simulink model "surgicalControl_Shared_memory_loop_2015b"  (R2015b)
settings: Solver=FixedStepAuto  SolverMode=SingleTasking  StartTime=0.0  StopTime=inf  FixedStep=1/100  RelTol=1e-3
libraries: dspsigops x9, simulink x3, matlabGenericSHM_Block x1
settings Model: Creator=daniel  LastModifiedBy=migf1
settings DataIOCC: LimitDataPoints=off
settings DebuggingCC: AllowSymbolicDim=on  SFUnexpectedBacktrackingDiag=error  SFNoUnconditionalDefaultTransitionDiag=error
settings ModelReferenceCC: PropagateSignalLabelsOutOfModel=on
settings GRTTargetCC: TargetLangStandard=C99 (ISO)
settings ConfigComp: CovMetricSettings=dwe  CovHtmlReporting=off  CovSaveCumulativeToWorkspaceVar=off  CovSaveSingleToWorkspaceVar=off  CovModelRefEnable=Off  CovExternalEMLEnable=on

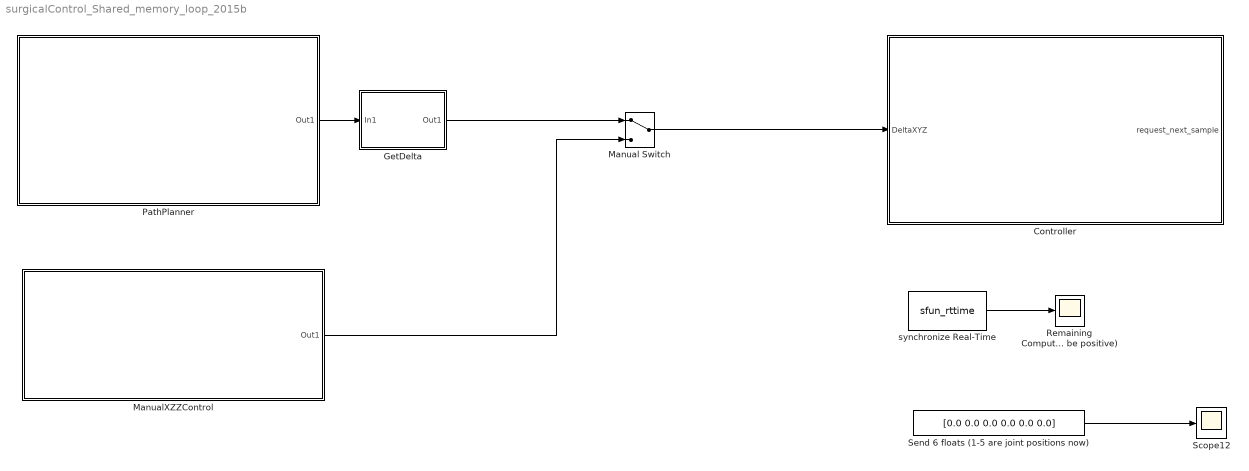
== system surgicalControl_Shared_memory_loop_2015b ==
  " GetDelta " : Subsystem
  Controller : Subsystem
  Manual Switch : ManualSwitch
  "ManualXZZControl " : Subsystem
  PathPlanner : Subsystem
  Remaining Computation Time (must be positive) : Scope
  Scope12 : Scope
  Send 6 floats (1-5 are joint positions now) : Constant  Value=[0.0 0.0 0.0 0.0 0.0 0.0]  OutDataTypeStr=single
  synchronize Real-Time : S-Function  FunctionName=sfun_rttime  Parameters=1  SFunctionDeploymentMode=off  EnableBusSupport=off
  wires:
  synchronize Real-Time/1 -> Remaining Computation Time (must be positive)/1
  Send 6 floats (1-5 are joint positions now)/1 -> Scope12/1
  Manual Switch/1 -> Controller/1(DeltaXYZ)
  PathPlanner/1(Out1) -> " GetDelta "/1(In1)
  "ManualXZZControl "/1(Out1) -> Manual Switch/2
  " GetDelta "/1(Out1) -> Manual Switch/1

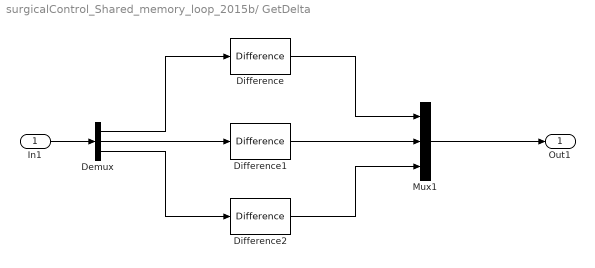
== system surgicalControl_Shared_memory_loop_2015b/ GetDelta  ==
  In1 : Inport
  Demux : Demux  Outputs=3
  Difference : simulink/Discrete/Difference  ICPrevInput=0  OutMin=[]  OutMax=[]  OutDataType=fixdt(1, 16)  OutScaling=2^-10  DoSatur=off
  Difference1 : simulink/Discrete/Difference  ICPrevInput=0  OutMin=[]  OutMax=[]  OutDataType=fixdt(1, 16)  OutScaling=2^-10  DoSatur=off
  Difference2 : simulink/Discrete/Difference  ICPrevInput=0  OutMin=[]  OutMax=[]  OutDataType=fixdt(1, 16)  OutScaling=2^-10  DoSatur=off
  Mux1 : Mux  Inputs=3
  Out1 : Outport
  wires:
  In1/1 -> Demux/1
  Demux/1 -> Difference/1
  Demux/2 -> Difference1/1
  Demux/3 -> Difference2/1
  Difference1/1 -> Mux1/2
  Difference/1 -> Mux1/1
  Difference2/1 -> Mux1/3
  Mux1/1 -> Out1/1

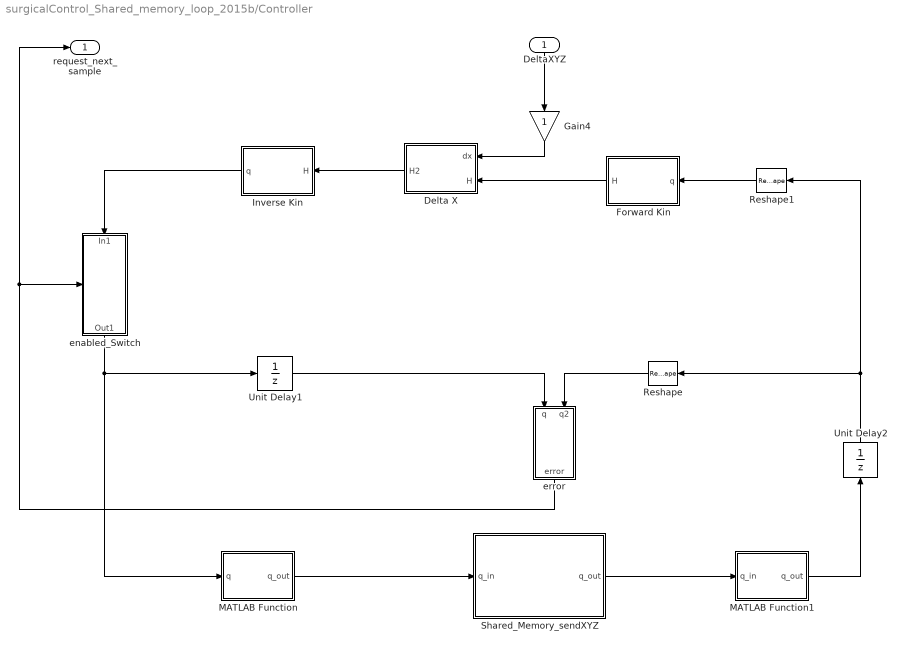
== system surgicalControl_Shared_memory_loop_2015b/Controller ==
  DeltaXYZ : Inport
  Delta X : MATLAB Function  TreatAsAtomicUnit=on
      settings: PermitHierarchicalResolution=ParametersOnly
  Forward Kin : MATLAB Function  TreatAsAtomicUnit=on
      settings: PermitHierarchicalResolution=ParametersOnly
  Gain4 : Gain
  Inverse Kin : MATLAB Function  TreatAsAtomicUnit=on
      settings: PermitHierarchicalResolution=ParametersOnly
  MATLAB Function : MATLAB Function  TreatAsAtomicUnit=on
      settings: PermitHierarchicalResolution=ParametersOnly
  MATLAB Function1 : MATLAB Function  TreatAsAtomicUnit=on
      settings: PermitHierarchicalResolution=ParametersOnly
  Reshape : Reshape
  Reshape1 : Reshape  OutputDimensionality=Customize  OutputDimensions=[1,6]
  Shared_Memory_sendXYZ : Subsystem  mask{ID1=4}
  Unit Delay1 : UnitDelay  InitialCondition=[0.0 0.0 0.0 0.0 0.0 0.0]  SampleTime=-1
  Unit Delay2 : UnitDelay  InitialCondition=[0.0 0.0 0.0 0.0 0.0 0.0]  SampleTime=-1
  "enabled_Switch " : Subsystem  TreatAsAtomicUnit=on
  error : MATLAB Function  TreatAsAtomicUnit=on
      settings: PermitHierarchicalResolution=ParametersOnly
  request_next_sample : Outport
  wires:
  Reshape/1 -> error/2(q2)
  MATLAB Function1/1(q_out) -> Unit Delay2/1
  Shared_Memory_sendXYZ/1(q_out) -> MATLAB Function1/1(q_in)
  Gain4/1 -> Delta X/1(dx)
  Forward Kin/1(H) -> Delta X/2(H)
  DeltaXYZ/1 -> Gain4/1
  Reshape1/1 -> Forward Kin/1(q)
  Unit Delay2/1 -> Reshape/1, Reshape1/1
  "enabled_Switch "/1(Out1) -> Unit Delay1/1, MATLAB Function/1(q)
  MATLAB Function/1(q_out) -> Shared_Memory_sendXYZ/1(q_in)
  error/1(error) -> request_next_sample/1, "enabled_Switch "/Enable
  Unit Delay1/1 -> error/1(q)
  Delta X/1(H2) -> Inverse Kin/1(H)
  Inverse Kin/1(q) -> "enabled_Switch "/1(In1)

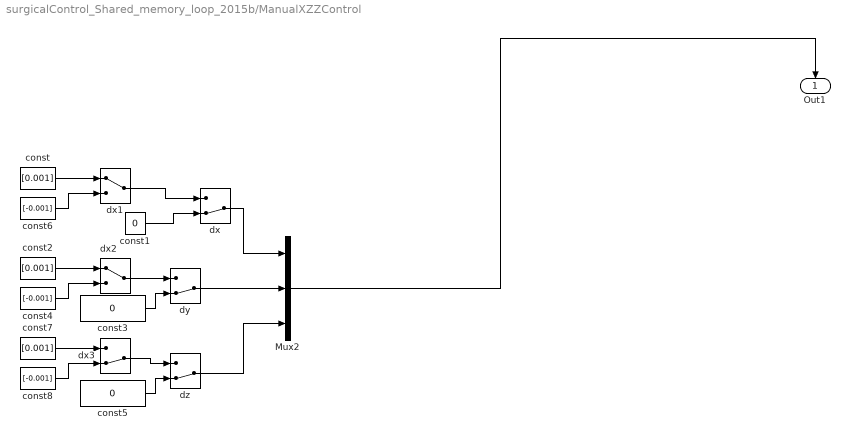
== system surgicalControl_Shared_memory_loop_2015b/ManualXZZControl  ==
  Mux2 : Mux  Inputs=3
  const : Constant  Value=[0.001]  OutDataTypeStr=single
  const1 : Constant  Value=0  OutDataTypeStr=single
  const2 : Constant  Value=[0.001]  OutDataTypeStr=single
  const3 : Constant  Value=0  OutDataTypeStr=single
  const4 : Constant  Value=[-0.001]  OutDataTypeStr=single
  const5 : Constant  Value=0  OutDataTypeStr=single
  const6 : Constant  Value=[-0.001]  OutDataTypeStr=single
  const7 : Constant  Value=[0.001]  OutDataTypeStr=single
  const8 : Constant  Value=[-0.001]  OutDataTypeStr=single
  dx : ManualSwitch  CurrentSetting=0
  dx1 : ManualSwitch
  dx2 : ManualSwitch
  dx3 : ManualSwitch  CurrentSetting=0
  dy : ManualSwitch  CurrentSetting=0
  dz : ManualSwitch  CurrentSetting=0
  Out1 : Outport
  wires:
  const/1 -> dx1/1
  const6/1 -> dx1/2
  const2/1 -> dx2/1
  dz/1 -> Mux2/3
  dx/1 -> Mux2/1
  dx2/1 -> dy/1
  dy/1 -> Mux2/2
  dx3/1 -> dz/1
  const5/1 -> dz/2
  Mux2/1 -> Out1/1
  const8/1 -> dx3/2
  const7/1 -> dx3/1
  const3/1 -> dy/2
  const1/1 -> dx/2
  dx1/1 -> dx/1
  const4/1 -> dx2/2

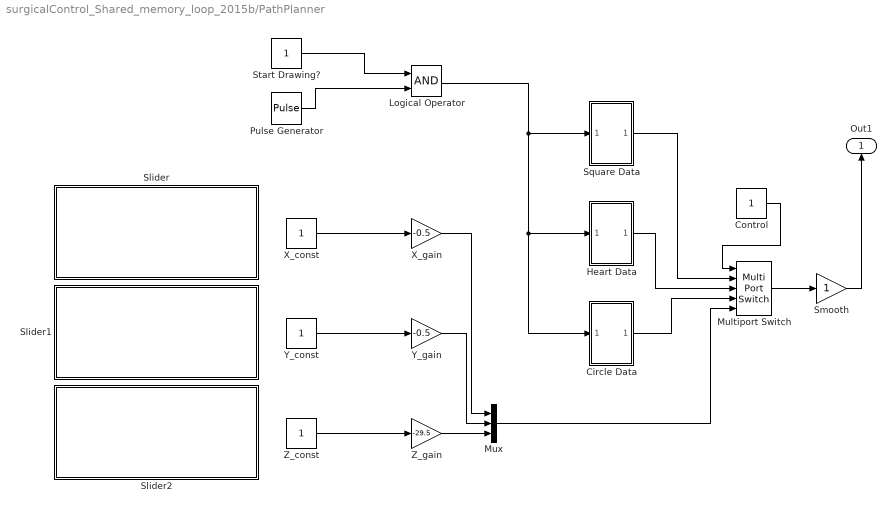
== system surgicalControl_Shared_memory_loop_2015b/PathPlanner ==
  " X_const " : Constant
  " Y_const" : Constant
  " Z_const" : Constant
  Circle Data : Subsystem
  "Control " : Constant
  Heart Data : Subsystem
  Logical Operator : Logic  AllPortsSameDT=off  OutDataTypeStr=boolean
  Multiport Switch : MultiPortSwitch  Inputs=4
  Mux : Mux  Inputs=3
  Pulse Generator : DiscretePulseGenerator  PulseType=Time based  Period=1  PulseWidth=20
  Slider : Subsystem  DialogController=hmiCreateDDGDialog  IsWebBlock=on  mask(MWDashboardBlock){webBlockId=4f94596f-dd6d-4e5e-bddc-7a8d913927f9, webBlockType=slider, ShowInLibBrowser=on, ShowInitialText=on, HMISrcModelName=surgicalControl_Shared_memory_loop_2015b}
      mask prompts: webBlockId "WebBlock Id"; webBlockType "WebBlock Type"; HMISrcModelName "Source Model"
      mask help: SimulinkHMI:dialogs:SliderDialogDesc
      mask Help: helpview([docroot '/mapfiles/simulink.map'], 'hmi_slider')
      mask Display:
      | if strcmp(get_param(bdroot(gcb),'BlockDiagramType'), 'library')
      |     image([(matlabroot) '/toolbox/simulink/hmi/icons/Slider.png']);
      | end
  Slider1 : Subsystem  DialogController=hmiCreateDDGDialog  IsWebBlock=on  mask(MWDashboardBlock){webBlockId=8aa996ad-7cd4-40fc-9a04-6a85939aea5d, webBlockType=slider, ShowInLibBrowser=on, ShowInitialText=on, HMISrcModelName=surgicalControl_Shared_memory_loop_2015b}
      mask prompts: webBlockId "WebBlock Id"; webBlockType "WebBlock Type"; HMISrcModelName "Source Model"
      mask help: SimulinkHMI:dialogs:SliderDialogDesc
      mask Help: helpview([docroot '/mapfiles/simulink.map'], 'hmi_slider')
      mask Display:
      | if strcmp(get_param(bdroot(gcb),'BlockDiagramType'), 'library')
      |     image([(matlabroot) '/toolbox/simulink/hmi/icons/Slider.png']);
      | end
  Slider2 : Subsystem  DialogController=hmiCreateDDGDialog  IsWebBlock=on  mask(MWDashboardBlock){webBlockId=1ddf6fd9-0225-4881-82ca-a25e179e2ab9, webBlockType=slider, ShowInLibBrowser=on, ShowInitialText=on, HMISrcModelName=surgicalControl_Shared_memory_loop_2015b}
      mask prompts: webBlockId "WebBlock Id"; webBlockType "WebBlock Type"; HMISrcModelName "Source Model"
      mask help: SimulinkHMI:dialogs:SliderDialogDesc
      mask Help: helpview([docroot '/mapfiles/simulink.map'], 'hmi_slider')
      mask Display:
      | if strcmp(get_param(bdroot(gcb),'BlockDiagramType'), 'library')
      |     image([(matlabroot) '/toolbox/simulink/hmi/icons/Slider.png']);
      | end
  Smooth : Gain
  "Square Data " : Subsystem
  Start Drawing? : Constant  SampleTime=1
  "X_gain " : Gain  Gain=-0.5
  "Y_gain " : Gain  Gain=-0.5
  Z_gain : Gain  Gain=-29.5
  Out1 : Outport
  wires:
  " Z_const"/1 -> Z_gain/1
  Z_gain/1 -> Mux/3
  "X_gain "/1 -> Mux/1
  "Control "/1 -> Multiport Switch/1
  Multiport Switch/1 -> Smooth/1
  " X_const "/1 -> "X_gain "/1
  Mux/1 -> Multiport Switch/5
  "Square Data "/1(xyz) -> Multiport Switch/2
  Smooth/1 -> Out1/1
  " Y_const"/1 -> "Y_gain "/1
  "Y_gain "/1 -> Mux/2
  Start Drawing?/1 -> Logical Operator/1
  Logical Operator/1 -> Heart Data/1(In1), Circle Data/1(In1), "Square Data "/1(In1)
  Heart Data/1(xyz) -> Multiport Switch/3
  Pulse Generator/1 -> Logical Operator/2
  Circle Data/1(xyz) -> Multiport Switch/4

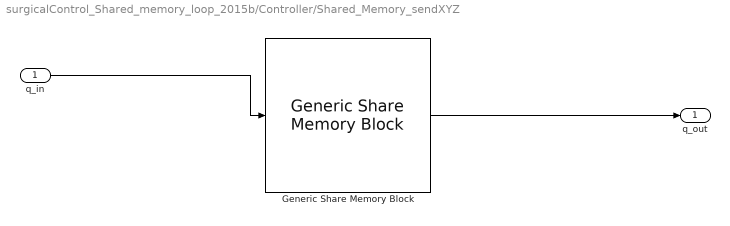
== system surgicalControl_Shared_memory_loop_2015b/Controller/Shared_Memory_sendXYZ ==
  q_in : Inport
  Generic Share Memory Block : matlabGenericSHM_Block/Generic Share Memory Block  nombre='EyeRob'  dispositivo=ID1  vecE=[6]  vecS=[6]  tipoE=['f']  tipoS=['f']
  q_out : Outport
  wires:
  q_in/1 -> Generic Share Memory Block/1
  Generic Share Memory Block/1 -> q_out/1

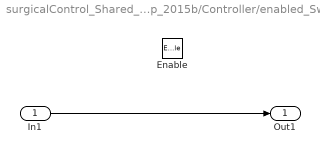
== system surgicalControl_Shared_memory_loop_2015b/Controller/enabled_Switch  ==
  In1 : Inport
  Enable : EnablePort
  Out1 : Outport
  wires:
  In1/1 -> Out1/1

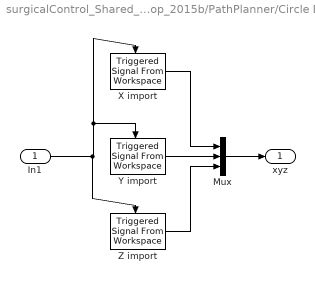
== system surgicalControl_Shared_memory_loop_2015b/PathPlanner/Circle Data ==
  In1 : Inport
  Mux : Mux  Inputs=3
  X import : dspsigops/Triggered Signal From Workspace  Signal=xs_circle  TriggerType=Falling edge  ic=0  SamplesPerFrame=1  OutputAfterFinalValue=Setting to zero  OutputFrames=off
  Y import : dspsigops/Triggered Signal From Workspace  Signal=ys_circle  TriggerType=Falling edge  ic=0  SamplesPerFrame=1  OutputAfterFinalValue=Setting to zero  OutputFrames=off
  Z import : dspsigops/Triggered Signal From Workspace  Signal=zs_circle  TriggerType=Falling edge  ic=0  SamplesPerFrame=1  OutputAfterFinalValue=Setting to zero  OutputFrames=off
  xyz : Outport
  wires:
  X import/1 -> Mux/1
  Z import/1 -> Mux/3
  Mux/1 -> xyz/1
  Y import/1 -> Mux/2
  In1/1 -> Z import/Trigger, X import/Trigger, Y import/Trigger

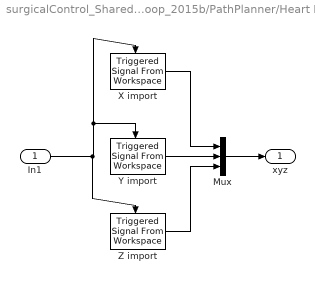
== system surgicalControl_Shared_memory_loop_2015b/PathPlanner/Heart Data ==
  In1 : Inport
  Mux : Mux  Inputs=3
  X import : dspsigops/Triggered Signal From Workspace  Signal=xs_heart  TriggerType=Falling edge  ic=0  SamplesPerFrame=1  OutputAfterFinalValue=Setting to zero  OutputFrames=off
  Y import : dspsigops/Triggered Signal From Workspace  Signal=ys_heart  TriggerType=Falling edge  ic=0  SamplesPerFrame=1  OutputAfterFinalValue=Setting to zero  OutputFrames=off
  Z import : dspsigops/Triggered Signal From Workspace  Signal=zs_heart  TriggerType=Falling edge  ic=0  SamplesPerFrame=1  OutputAfterFinalValue=Setting to zero  OutputFrames=off
  xyz : Outport
  wires:
  X import/1 -> Mux/1
  Z import/1 -> Mux/3
  Mux/1 -> xyz/1
  Y import/1 -> Mux/2
  In1/1 -> Z import/Trigger, X import/Trigger, Y import/Trigger

== system surgicalControl_Shared_memory_loop_2015b/PathPlanner/Slider ==

== system surgicalControl_Shared_memory_loop_2015b/PathPlanner/Slider1 ==

== system surgicalControl_Shared_memory_loop_2015b/PathPlanner/Slider2 ==

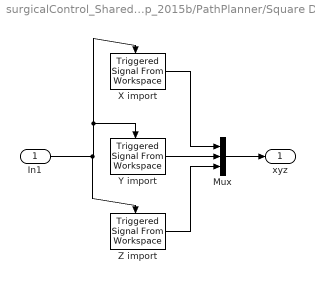
== system surgicalControl_Shared_memory_loop_2015b/PathPlanner/Square Data  ==
  In1 : Inport
  Mux : Mux  Inputs=3
  X import : dspsigops/Triggered Signal From Workspace  Signal=xs_square  TriggerType=Falling edge  ic=0  SamplesPerFrame=1  OutputAfterFinalValue=Setting to zero  OutputFrames=off
  Y import : dspsigops/Triggered Signal From Workspace  Signal=ys_square  TriggerType=Falling edge  ic=0  SamplesPerFrame=1  OutputAfterFinalValue=Setting to zero  OutputFrames=off
  Z import : dspsigops/Triggered Signal From Workspace  Signal=zs_square  TriggerType=Falling edge  ic=0  SamplesPerFrame=1  OutputAfterFinalValue=Setting to zero  OutputFrames=off
  xyz : Outport
  wires:
  X import/1 -> Mux/1
  Z import/1 -> Mux/3
  Mux/1 -> xyz/1
  Y import/1 -> Mux/2
  In1/1 -> Z import/Trigger, X import/Trigger, Y import/Trigger

== matlab function surgicalControl_Shared_memory_loop_2015b/Controller/Forward Kin ==
  data: q input; H output
function H = fcn(q)
H = fKin(q);

== matlab function surgicalControl_Shared_memory_loop_2015b/Controller/Delta X ==
  data: dx input; H input; H2 output
function H2 = fcn(dx,H)
H2 = H;
H2(1,4)=H2(1,4)+dx(3,1);
H2(2,4)=H2(2,4)+dx(2,1);
H2(3,4)=H2(3,4)+dx(1,1);
end

== matlab function surgicalControl_Shared_memory_loop_2015b/Controller/error ==
  data: q input; error output; q2 input
function error = fcn(q,q2)
H1 = fKin(q');
H2 = fKin(q2');
H=H1-H2;
error=(norm(H(1:3,4)')<0.001);
end

== matlab function surgicalControl_Shared_memory_loop_2015b/Controller/MATLAB Function ==
  data: q input size=[1 6]; q_out output size=[1 6]
function q_out = correctForPrismatic(q)
%#codegen
 if iscolumn(q)
       q = q';
 end
q_out=zeros(1, 6,'single');

q1=q(1,1);
q2=q(1,2);
q3=q(1,3);
q4=q(1,4);
q2_temp= getL2(q1,q2);
q4_temp= getL1(q3,q4);

% end


q_out(1,1) = q1+0.0049;
q_out(1,2) = q2_temp;
q_out(1,3) = q3;
q_out(1,4) = q4_temp;
q_out(1,5) = q(1,5);
q_out(1,6) = q(1,6);
end

== matlab function surgicalControl_Shared_memory_loop_2015b/Controller/MATLAB Function1 ==
  data: q_in input size=[1 6]; q_out output size=[1 6]
function q_out = recorrectForPrismatic(q_in)
%#codegen
q=q_in;
q_out=zeros(1, 6,'double');
d= 17e-3;

q1=q(1,1)-0.0049;
q2=q(1,2);
q3=q(1,3);
q4=q(1,4);
q2_temp= atan((q2-q1)/d);
q4_temp= atan((q3-q4)/d); 

% end
%q_out=[q1,q2_temp,q3,q4_temp,q(1,5),q(1,6)];

q_out(1,1) = q1;
q_out(1,2) = q2_temp;
q_out(1,3) = q3;
q_out(1,4) = q4_temp;
q_out(1,5) = q(1,5);
q_out(1,6) = q(1,6);
%q_out=round(q_out*1000)/1000;
end

== matlab function surgicalControl_Shared_memory_loop_2015b/Controller/Inverse Kin ==
  data: H input; q output
function q = fcn(H)

%q = round(IK(H)'*1000)/1000;
q = IK(H)';
